simulink library "LevelDetectorLib"  (R2022b)
settings: Solver=VariableStepAuto  StartTime=0.0  StopTime=10.0  RelTol=1e-3
libraries: LevelDetectorLibBtc x1
settings Model: Creator=db1045444  LastModifiedBy=kl13806
settings SolverCC: AlgebraicLoopSolver=TrustRegion
settings DebuggingCC: UnconnectedInputMsg=warning  UnconnectedOutputMsg=warning  UnconnectedLineMsg=warning  SFMachineParentedDataDiag=warning  ArithmeticOperatorsInVariantConditions=warning
settings ModelReferenceCC: EnableRefExpFcnMdlSchedulingChecks=on
settings SFSimCC: CustomCodeUndefinedFunction=UseInterfaceOnly
settings RTWCC: DLArmComputeVersion=19.05

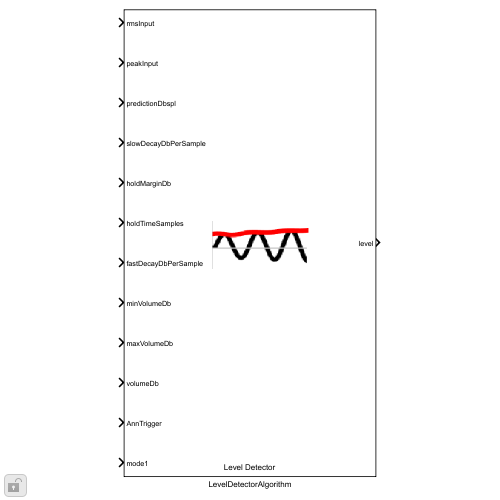
[thumbnail: Simulink's stored preview of the top-level diagram]
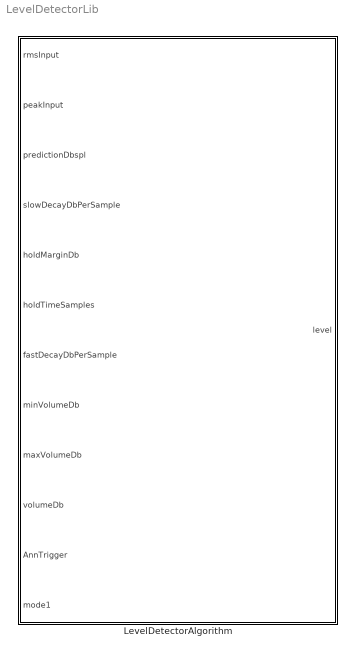
== system LevelDetectorLib ==
  LevelDetectorAlgorithm : Subsystem  mask(Bose Level Detector Algorithm){MaskAnnTriggerThreshold=single(0.5), MaskSuperFastDecayMultiplier=single(3.0)}
      mask prompts: MaskAnnTriggerThreshold "Announcement trigger threshold"; MaskSuperFastDecayMultiplier "Announcement super fast decay multiplier"
      mask help: Computes signal level in dB using a combination of the attack, slow decay, hold and fast decay phases. Check the Help menu for a description of the parameters.
      mask init:
      | blkh = gcbh;
      | % Copy discrete mask parameters into a classdef object
      | InnerLinkConfig = LevelDetectorConfig;
      | InnerLinkConfig.AnnTriggerThreshold = MaskAnnTriggerThreshold;
      | InnerLinkConfig.SuperFastDecayMultiplier = MaskSuperFastDecayMultiplier;
      mask Help:
      | Detects signal level in dB using a combination of the attack, slow decay, hold and fast decay phases.
      | - 'mode' determines which input is used (0 = RMS or 1 = Peak input)
      | - Decay parameters are tunable
      |   - holdTimeSamples and holdMarginDb are taken as positive values
      |   - slowDecayDbPerSample and fastDecayDbPerSample are taken as negative values
      |   - slowDecayDbPerSample, fastDecayDbPerSample and holdTimeSamples are to be provided in #samples. So, if they are originally defined differently (for example- decay in dB or hold time in seconds), a "tune translation" (or similar) needs to occur to convert them to the corresponding #samples based on the sampling frequency.
      | - 'Announcement super fast decay coefficient' determines how fast we want the level to drop in case there is an announcement
      | - 'AnnTrigger' refers to the current value of the announcement trigger. When this value is greater than the 'Announcement threshold', the 'super fast decay coefficient' will be applied to the audio.
      mask Display:
      | img = imread('LevelDetectorIcon.PNG');
      | [w, h, ~] = size(img);
      | 
      | % retrieve the block's pixel size
      | pos = get(gcbh,'position');
      | bw = pos(3) - pos(1);
      | bh = pos(4) - pos(2);
      | 
      | xAdj = bw/2 - w/2 +30;
      | yAdj = bh/2 - h/2;
      | image('LevelDetectorIcon.PNG', [xAdj, yAdj, w, h]);
      | 
      | % place feature name text
      | text(bw*0.5, 0, ['Level Detector' '\n\n'], 'horizontalAlignment', 'center');

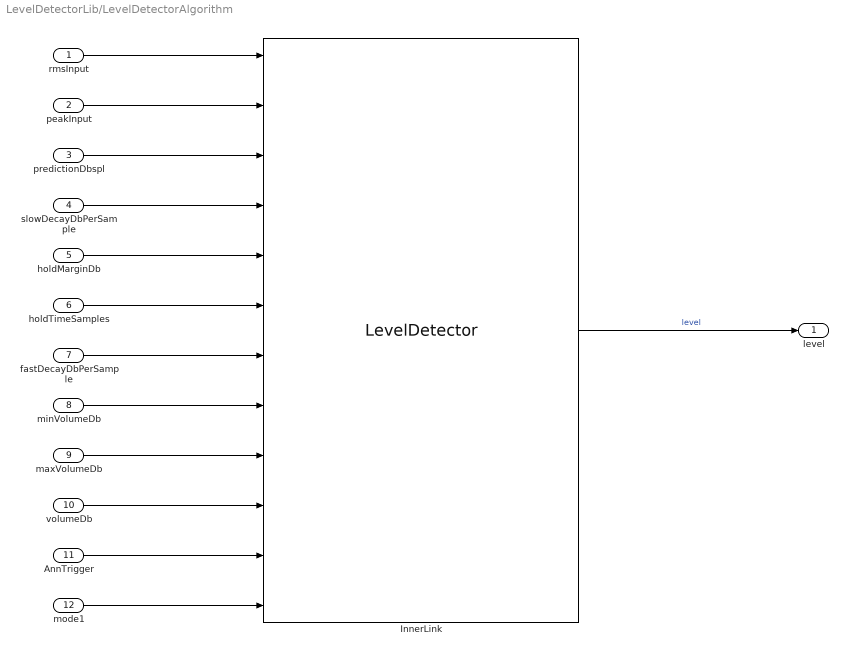
== system LevelDetectorLib/LevelDetectorAlgorithm ==
  rmsInput : Inport
  peakInput : Inport  Port=2
  predictionDbspl : Inport  Port=3
  slowDecayDbPerSample : Inport  Port=4
  holdMarginDb : Inport  Port=5
  holdTimeSamples : Inport  Port=6
  fastDecayDbPerSample : Inport  Port=7
  minVolumeDb : Inport  Port=8
  maxVolumeDb : Inport  Port=9
  volumeDb : Inport  Port=10
  AnnTrigger : Inport  Port=11
  mode1 : Inport  Port=12
  InnerLink : LevelDetectorLibBtc/LevelDetector  Config=InnerLinkConfig
      settings: SourceProductName=Bose Blocklib
  level : Outport
  wires:
  maxVolumeDb/1 -> InnerLink/9
  predictionDbspl/1 -> InnerLink/3
  holdMarginDb/1 -> InnerLink/5
  slowDecayDbPerSample/1 -> InnerLink/4
  volumeDb/1 -> InnerLink/10
  holdTimeSamples/1 -> InnerLink/6
  minVolumeDb/1 -> InnerLink/8
  fastDecayDbPerSample/1 -> InnerLink/7
  AnnTrigger/1 -> InnerLink/11
  mode1/1 -> InnerLink/12
  rmsInput/1 -> InnerLink/1
  InnerLink/1 -> level/1  "level"
  peakInput/1 -> InnerLink/2
